simulink model "NDT_Localization"  (R2022a)
settings: Solver=FixedStepAuto  StartTime=0.0  StopTime=10.0  RelTol=1e-3
model workspace (MAT data in the model file):
  SL_ROS_VariableLengthArrays_MaxSizes : object (value not decoded)
undefined symbols (not defined in the file or in its folder): null
libraries: ros2lib x9, robotlib x8, simulink x1
(part 9 of 12)

== system NDT_Localization/observation_callback/check_localizer/If Action Subsystem/register_measurement_impl/If Action Subsystem/If Action Subsystem/solve/If Action Subsystem1/For Iterator Subsystem/compute_next_step/If Action Subsystem1/For Iterator Subsystem/If Action Subsystem/If Action Subsystem3/If Action Subsystem/f_l/gradient_angle ==
  params : Inport
  Add : Sum
  Add{1,3..5,7} (5 alike) : Sum  Inputs=+-
  Add2 : Sum
  Add6 : Sum
  Bus Selector : BusSelector  OutputSignals=cx,sx,cy,sy,cz,sz
  Constant : Constant  Value=0.0
  Constant1 : Constant  Value=0.0
  Constant2 : Constant  Value=0.0
  Gain{,1..3} (4 alike) : Gain  Gain=-1
  Product{,2,4..5,7,9..11,14,17..20,22,24,27} (16 alike) : Product
  Product{1,3,6,8,12..13,15..16,21,23,25..26} (12 alike) : Product  Inputs=3
  ga_a : MATLAB Function  TreatAsAtomicUnit=on
  ga_b : MATLAB Function  TreatAsAtomicUnit=on
  ga_c : MATLAB Function  TreatAsAtomicUnit=on
  ga_d : MATLAB Function  TreatAsAtomicUnit=on
  ga_e : MATLAB Function  TreatAsAtomicUnit=on
  ga_f : MATLAB Function  TreatAsAtomicUnit=on
  ga_g : MATLAB Function  TreatAsAtomicUnit=on
  ga_h : MATLAB Function  TreatAsAtomicUnit=on
  ga_a_out : Outport
  ga_b_out : Outport  Port=2
  ga_c_out : Outport  Port=3
  ga_d_out : Outport  Port=4
  ga_e_out : Outport  Port=5
  ga_f_out : Outport  Port=6
  ga_g_out : Outport  Port=7
  ga_h_out : Outport  Port=8
  wires:
  params/1 -> Bus Selector/1
  Bus Selector/1 -> Product1/1, Product16/1, Product25/1, Product26/1, Product20/1, Product7/1, Product5/1, Product3/1, Gain/1  "<cx>"
  Bus Selector/2 -> Product6/1, Product12/1, Product14/1, Product21/1, Product23/1, Product27/1, Product24/1, Product8/1, Gain1/1  "<sx>"
  Bus Selector/3 -> Product12/2, Product13/2, Product15/2, Product16/2, ga_c/3(z), Product9/2, Product4/2, Gain2/1  "<cy>"
  Bus Selector/4 -> Product11/1, Product14/2, Product17/2, Product21/2, Product25/2, Product26/2, Product23/2, Product8/2, Product6/2, Product3/2, Product1/2, Gain3/1  "<cx>"
  Bus Selector/5 -> Product6/3, Product10/2, Product12/3, Product15/3, Product19/2, Product20/2, Product23/3, Product26/3, Product24/2, Product7/2, Product2/2, Product1/3  "<cx>"
  Bus Selector/6 -> Product11/2, Product13/3, Product16/3, Product18/2, Product21/3, Product22/2, Product25/3, Product27/2, Product8/3, Product5/2, Product3/3, Product/2  "<cx>"
  Gain1/1 -> Product13/1, Product9/1, Product2/1, Product/1
  Product/1 -> Add/1
  Product1/1 -> Add/2
  Product2/1 -> Add1/1
  Add/1 -> ga_a/1(x)
  Add1/1 -> ga_a/2(y)
  Gain/1 -> Product15/1, Product17/1, Product22/1, Product4/1
  Product4/1 -> ga_a/3(z)
  Product3/1 -> Add1/2
  Product6/1 -> Add2/2
  Product7/1 -> Add3/1
  Product8/1 -> Add3/2
  Product5/1 -> Add2/1
  Add2/1 -> ga_b/1(x)
  Product9/1 -> ga_b/3(z)
  Add3/1 -> ga_b/2(y)
  Product11/1 -> ga_c/2(y)
  Product10/1 -> ga_c/1(x)
  Gain2/1 -> Product18/1, Product19/1
  Gain3/1 -> Product10/1
  Product13/1 -> ga_d/2(y)
  Product12/1 -> ga_d/1(x)
  Product14/1 -> ga_d/3(z)
  Product19/1 -> ga_f/2(y)
  Constant/1 -> ga_f/3(z)
  Product18/1 -> ga_f/1(x)
  Product16/1 -> ga_e/2(y)
  Product17/1 -> ga_e/3(z)
  Product15/1 -> ga_e/1(x)
  Product21/1 -> Add4/2
  Product22/1 -> Add5/1
  Product23/1 -> Add5/2
  Product20/1 -> Add4/1
  Add5/1 -> ga_g/2(y)
  Product25/1 -> Add6/2
  Product26/1 -> Add7/1
  Product27/1 -> Add7/2
  Product24/1 -> Add6/1
  Constant1/1 -> ga_g/3(z)
  Add4/1 -> ga_g/1(x)
  Add7/1 -> ga_h/2(y)
  Add6/1 -> ga_h/1(x)
  Constant2/1 -> ga_h/3(z)
  ga_a/1(out) -> ga_a_out/1  "a"
  ga_b/1(out) -> ga_b_out/1  "b"
  ga_c/1(out) -> ga_c_out/1  "c"
  ga_d/1(out) -> ga_d_out/1  "d"
  ga_e/1(out) -> ga_e_out/1  "e"
  ga_f/1(out) -> ga_f_out/1  "f"
  ga_g/1(out) -> ga_g_out/1  "g"
  ga_h/1(out) -> ga_h_out/1  "h"

== system NDT_Localization/observation_callback/check_localizer/If Action Subsystem/register_measurement_impl/If Action Subsystem/If Action Subsystem/solve/If Action Subsystem1/For Iterator Subsystem/compute_next_step/If Action Subsystem1/For Iterator Subsystem/If Action Subsystem/If Action Subsystem3/If Action Subsystem/f_u/For Iterator Subsystem ==
  data : Inport
  myu : Inport  Port=2
  sigma : Inport  Port=3
  outlier_ratio : Inport  Port=4
  voxel_size_x : Inport  Port=5
  voxel_size_y : Inport  Port=6
  voxel_size_z : Inport  Port=7
  set_jacobian : Inport  Port=8
  set_gradient : Inport  Port=9
  Affine : MATLAB Function  TreatAsAtomicUnit=on
  Delay : Delay  DelayLength=1
  For Iterator : ForIterator  IterationSource=external
  MATLAB Function : MATLAB Function  TreatAsAtomicUnit=on
  Width : Width
  gradient_jaco : Subsystem
  make_c_param : Subsystem
  make_d_param : Subsystem
  score : Subsystem
  score_out : Outport
  jacobian_out : Outport  Port=2
  wires:
  make_c_param/1(c1) -> make_d_param/1(c1)
  voxel_size_z/1 -> make_c_param/4(voxel_size_z)
  outlier_ratio/1 -> make_c_param/1(outlier_ratio)
  make_d_param/2(d2) -> gradient_jaco/9(d2), score/6(d2)
  voxel_size_y/1 -> make_c_param/3(voxel_size_y)
  make_c_param/2(c2) -> make_d_param/2(c2)
  voxel_size_x/1 -> make_c_param/2(voxel_size_x)
  make_d_param/1(d1) -> score/5(d1), gradient_jaco/8(d1)
  Width/1 -> For Iterator/1
  For Iterator/1 -> gradient_jaco/3(index), MATLAB Function/2(index)
  MATLAB Function/1(pt) -> Affine/1(u)
  Affine/1(out) -> score/4(x), gradient_jaco/4(data)
  sigma/1 -> score/2(sigma), gradient_jaco/5(sigma)
  myu/1 -> gradient_jaco/6(myu), score/3(myu)
  score/1(p) -> score_out/1, Delay/1
  Delay/1 -> score/1(score)
  set_jacobian/1 -> gradient_jaco/1(set_jacobian)
  gradient_jaco/1(Out1) -> jacobian_out/1
  set_gradient/1 -> gradient_jaco/2(set_gradient)
  data/1 -> gradient_jaco/7(x), MATLAB Function/1(data), Width/1

== system NDT_Localization/observation_callback/check_localizer/If Action Subsystem/register_measurement_impl/If Action Subsystem/If Action Subsystem/solve/If Action Subsystem1/For Iterator Subsystem/compute_next_step/If Action Subsystem1/For Iterator Subsystem/If Action Subsystem/If Action Subsystem3/If Action Subsystem/f_u/angle_params ==
  pose : Inport
  Bus Creator : BusCreator  Inputs=6
  If : If  NumInputs=2  IfExpression=u1 > u2
  If Action Subsystem : Subsystem  TreatAsAtomicUnit=on
  If Action Subsystem1 : Subsystem  TreatAsAtomicUnit=on
  If Action Subsystem2 : Subsystem  TreatAsAtomicUnit=on
  If Action Subsystem3 : Subsystem  TreatAsAtomicUnit=on
  If Action Subsystem4 : Subsystem  TreatAsAtomicUnit=on
  If Action Subsystem5 : Subsystem  TreatAsAtomicUnit=on
  If1 : If  NumInputs=2  IfExpression=u1 > u2
  If2 : If  NumInputs=2  IfExpression=u1 > u2
  MATLAB Function : MATLAB Function  TreatAsAtomicUnit=on
  Merge{,1..5} (6 alike) : Merge
  approx_thresh : Constant  Value=0.00010
  params : Outport
  wires:
  pose/1 -> MATLAB Function/1(u)
  MATLAB Function/1(x) -> If/2, If Action Subsystem1/1(x)
  MATLAB Function/3(z) -> If2/2, If Action Subsystem5/1(z)
  MATLAB Function/2(y) -> If Action Subsystem3/1(y), If1/2
  If Action Subsystem1/1(Out1) -> Merge/2
  If Action Subsystem1/2(Out2) -> Merge1/2
  If Action Subsystem3/1(Out1) -> Merge2/2
  If Action Subsystem3/2(Out2) -> Merge3/2
  If Action Subsystem5/1(Out1) -> Merge4/2
  If Action Subsystem5/2(Out2) -> Merge5/2
  approx_thresh/1 -> If2/1, If1/1, If/1
  If/1 -> If Action Subsystem/Action
  If/2 -> If Action Subsystem1/Action
  If1/1 -> If Action Subsystem2/Action
  If1/2 -> If Action Subsystem3/Action
  If2/2 -> If Action Subsystem5/Action
  If2/1 -> If Action Subsystem4/Action
  If Action Subsystem/1(Out1) -> Merge/1
  If Action Subsystem/2(Out2) -> Merge1/1
  If Action Subsystem2/1(Out1) -> Merge2/1
  If Action Subsystem2/2(Out2) -> Merge3/1
  If Action Subsystem4/1(Out1) -> Merge4/1
  If Action Subsystem4/2(Out2) -> Merge5/1
  Bus Creator/1 -> params/1
  Merge/1 -> Bus Creator/1  "cx"
  Merge1/1 -> Bus Creator/2  "sx"
  Merge2/1 -> Bus Creator/3  "cy"
  Merge3/1 -> Bus Creator/4  "sy"
  Merge4/1 -> Bus Creator/5  "cz"
  Merge5/1 -> Bus Creator/6  "sz"

== system NDT_Localization/observation_callback/check_localizer/If Action Subsystem/register_measurement_impl/If Action Subsystem/If Action Subsystem/solve/If Action Subsystem1/For Iterator Subsystem/compute_next_step/If Action Subsystem1/For Iterator Subsystem/If Action Subsystem/If Action Subsystem3/If Action Subsystem/f_u/gradient_angle ==
  params : Inport
  Add : Sum
  Add{1,3..5,7} (5 alike) : Sum  Inputs=+-
  Add2 : Sum
  Add6 : Sum
  Bus Selector : BusSelector  OutputSignals=cx,sx,cy,sy,cz,sz
  Constant : Constant  Value=0.0
  Constant1 : Constant  Value=0.0
  Constant2 : Constant  Value=0.0
  Gain{,1..3} (4 alike) : Gain  Gain=-1
  Product{,2,4..5,7,9..11,14,17..20,22,24,27} (16 alike) : Product
  Product{1,3,6,8,12..13,15..16,21,23,25..26} (12 alike) : Product  Inputs=3
  ga_a : MATLAB Function  TreatAsAtomicUnit=on
  ga_b : MATLAB Function  TreatAsAtomicUnit=on
  ga_c : MATLAB Function  TreatAsAtomicUnit=on
  ga_d : MATLAB Function  TreatAsAtomicUnit=on
  ga_e : MATLAB Function  TreatAsAtomicUnit=on
  ga_f : MATLAB Function  TreatAsAtomicUnit=on
  ga_g : MATLAB Function  TreatAsAtomicUnit=on
  ga_h : MATLAB Function  TreatAsAtomicUnit=on
  ga_a_out : Outport
  ga_b_out : Outport  Port=2
  ga_c_out : Outport  Port=3
  ga_d_out : Outport  Port=4
  ga_e_out : Outport  Port=5
  ga_f_out : Outport  Port=6
  ga_g_out : Outport  Port=7
  ga_h_out : Outport  Port=8
  wires:
  params/1 -> Bus Selector/1
  Bus Selector/1 -> Product1/1, Product16/1, Product25/1, Product26/1, Product20/1, Product7/1, Product5/1, Product3/1, Gain/1  "<cx>"
  Bus Selector/2 -> Product6/1, Product12/1, Product14/1, Product21/1, Product23/1, Product27/1, Product24/1, Product8/1, Gain1/1  "<sx>"
  Bus Selector/3 -> Product12/2, Product13/2, Product15/2, Product16/2, ga_c/3(z), Product9/2, Product4/2, Gain2/1  "<cy>"
  Bus Selector/4 -> Product11/1, Product14/2, Product17/2, Product21/2, Product25/2, Product26/2, Product23/2, Product8/2, Product6/2, Product3/2, Product1/2, Gain3/1  "<cx>"
  Bus Selector/5 -> Product6/3, Product10/2, Product12/3, Product15/3, Product19/2, Product20/2, Product23/3, Product26/3, Product24/2, Product7/2, Product2/2, Product1/3  "<cx>"
  Bus Selector/6 -> Product11/2, Product13/3, Product16/3, Product18/2, Product21/3, Product22/2, Product25/3, Product27/2, Product8/3, Product5/2, Product3/3, Product/2  "<cx>"
  Gain1/1 -> Product13/1, Product9/1, Product2/1, Product/1
  Product/1 -> Add/1
  Product1/1 -> Add/2
  Product2/1 -> Add1/1
  Add/1 -> ga_a/1(x)
  Add1/1 -> ga_a/2(y)
  Gain/1 -> Product15/1, Product17/1, Product22/1, Product4/1
  Product4/1 -> ga_a/3(z)
  Product3/1 -> Add1/2
  Product6/1 -> Add2/2
  Product7/1 -> Add3/1
  Product8/1 -> Add3/2
  Product5/1 -> Add2/1
  Add2/1 -> ga_b/1(x)
  Product9/1 -> ga_b/3(z)
  Add3/1 -> ga_b/2(y)
  Product11/1 -> ga_c/2(y)
  Product10/1 -> ga_c/1(x)
  Gain2/1 -> Product18/1, Product19/1
  Gain3/1 -> Product10/1
  Product13/1 -> ga_d/2(y)
  Product12/1 -> ga_d/1(x)
  Product14/1 -> ga_d/3(z)
  Product19/1 -> ga_f/2(y)
  Constant/1 -> ga_f/3(z)
  Product18/1 -> ga_f/1(x)
  Product16/1 -> ga_e/2(y)
  Product17/1 -> ga_e/3(z)
  Product15/1 -> ga_e/1(x)
  Product21/1 -> Add4/2
  Product22/1 -> Add5/1
  Product23/1 -> Add5/2
  Product20/1 -> Add4/1
  Add5/1 -> ga_g/2(y)
  Product25/1 -> Add6/2
  Product26/1 -> Add7/1
  Product27/1 -> Add7/2
  Product24/1 -> Add6/1
  Constant1/1 -> ga_g/3(z)
  Add4/1 -> ga_g/1(x)
  Add7/1 -> ga_h/2(y)
  Add6/1 -> ga_h/1(x)
  Constant2/1 -> ga_h/3(z)
  ga_a/1(out) -> ga_a_out/1  "a"
  ga_b/1(out) -> ga_b_out/1  "b"
  ga_c/1(out) -> ga_c_out/1  "c"
  ga_d/1(out) -> ga_d_out/1  "d"
  ga_e/1(out) -> ga_e_out/1  "e"
  ga_f/1(out) -> ga_f_out/1  "f"
  ga_g/1(out) -> ga_g_out/1  "g"
  ga_h/1(out) -> ga_h_out/1  "h"

== system NDT_Localization/observation_callback/check_localizer/If Action Subsystem/register_measurement_impl/If Action Subsystem/If Action Subsystem/solve/If Action Subsystem1/For Iterator Subsystem/compute_next_step/If Action Subsystem1/For Iterator Subsystem/If Action Subsystem/If Action Subsystem3/phi_t/For Iterator Subsystem/gradient_jaco ==
  set_jacobian : Inport
  set_gradient : Inport  Port=2
  index : Inport  Port=3
  data : Inport  Port=4
  sigma : Inport  Port=5
  myu : Inport  Port=6
  x : Inport  Port=7
  d1 : Inport  Port=8
  d2 : Inport  Port=9
  Add : Sum  Inputs=+-
  Constant : Constant  Value=-2
  Divide1 : Product  Inputs=*/
  Math Function : Math
  Math Function1 : Math  Operator=transpose
  Math Function2 : Math  Operator=reciprocal
  Product : Product  Inputs=4
  Product1 : Product  Inputs=3  Multiplication=Matrix(*)
  Product2 : Product
  Product3 : Product
  Product4 : Product  Multiplication=Matrix(*)
  gradient_col : MATLAB Function  TreatAsAtomicUnit=on
  jaco_add : MATLAB Function  TreatAsAtomicUnit=on
  Out1 : Outport
  wires:
  myu/1 -> Add/2
  Constant/1 -> Divide1/2
  Math Function1/1 -> Product1/1
  Divide1/1 -> Product2/1
  d2/1 -> Divide1/1, Product/3  "d2"
  Math Function2/1 -> Product3/2, Product1/2  "inv_cov"
  Product1/1 -> Product2/2
  d1/1 -> Product/2  "d1"
  x/1 -> Add/1
  Math Function/1 -> Product/4
  Product2/1 -> Math Function/1
  Add/1 -> Product1/3, Math Function1/1  "x-myu"
  sigma/1 -> Math Function2/1
  Product/1 -> jaco_add/3(num)
  index/1 -> jaco_add/2(index), gradient_col/1(index)
  jaco_add/1(jacobian) -> Out1/1
  set_jacobian/1 -> jaco_add/1("jacobian ")
  set_gradient/1 -> gradient_col/2(gradient)
  gradient_col/1(y) -> Product3/1
  data/1 -> Product4/1
  Product3/1 -> Product4/2
  Product4/1 -> Product/1

== system NDT_Localization/observation_callback/check_localizer/If Action Subsystem/register_measurement_impl/If Action Subsystem/If Action Subsystem/solve/If Action Subsystem1/For Iterator Subsystem/compute_next_step/If Action Subsystem1/For Iterator Subsystem/If Action Subsystem/If Action Subsystem3/phi_t/For Iterator Subsystem/make_c_param ==
  outlier_ratio : Inport
  voxel_size_x : Inport  Port=2
  voxel_size_y : Inport  Port=3
  voxel_size_z : Inport  Port=4
  Constant : Constant
  Divide : Product  Inputs=*/
  Gain : Gain  Gain=10
  Product : Product  Inputs=3
  Subtract : Sum  Inputs=+-
  c1 : Outport
  c2 : Outport  Port=2
  wires:
  Constant/1 -> Subtract/1
  outlier_ratio/1 -> Divide/1, Subtract/2
  Subtract/1 -> Gain/1
  Gain/1 -> c1/1
  Product/1 -> Divide/2
  Divide/1 -> c2/1
  voxel_size_y/1 -> Product/2
  voxel_size_z/1 -> Product/3
  voxel_size_x/1 -> Product/1

== system NDT_Localization/observation_callback/check_localizer/If Action Subsystem/register_measurement_impl/If Action Subsystem/If Action Subsystem/solve/If Action Subsystem1/For Iterator Subsystem/compute_next_step/If Action Subsystem1/For Iterator Subsystem/If Action Subsystem/If Action Subsystem3/phi_t/For Iterator Subsystem/make_d_param ==
  c1 : Inport
  c2 : Inport  Port=2
  Add1 : Sum
  Add2 : Sum  Inputs=-+
  Add3 : Sum
  Add4 : Sum  Inputs=+-
  Constant : Constant  Value=-2
  Constant1 : Constant  Value=-0.5
  Divide : Product  Inputs=*/
  Math Function{3..4,6..7} (4 alike) : Math  Operator=log
  Math Function5 : Math
  Product3 : Product
  Product4 : Product
  d1 : Outport
  d2 : Outport  Port=2
  wires:
  Add2/1 -> Divide/2, d1/1  "d1"
  Math Function4/1 -> Add4/1, Add2/2  "-d3"
  Product4/1 -> Add3/1
  Add3/1 -> Math Function6/1
  c1/1 -> Product4/1, Add1/1
  Constant/1 -> Product3/2
  Constant1/1 -> Math Function5/1
  Product3/1 -> d2/1  "d2"
  Math Function5/1 -> Product4/2
  Math Function7/1 -> Product3/1
  Divide/1 -> Math Function7/1
  Math Function6/1 -> Add4/2
  c2/1 -> Add3/2, Math Function4/1, Add1/2
  Add4/1 -> Divide/1
  Add1/1 -> Math Function3/1
  Math Function3/1 -> Add2/1

== system NDT_Localization/observation_callback/check_localizer/If Action Subsystem/register_measurement_impl/If Action Subsystem/If Action Subsystem/solve/If Action Subsystem1/For Iterator Subsystem/compute_next_step/If Action Subsystem1/For Iterator Subsystem/If Action Subsystem/If Action Subsystem3/phi_t/For Iterator Subsystem/score ==
  score : Inport
  sigma : Inport  Port=2
  myu : Inport  Port=3
  x : Inport  Port=4
  d1 : Inport  Port=5
  d2 : Inport  Port=6
  Add : Sum  Inputs=+-
  Add1 : Sum
  Constant : Constant  Value=-2
  Divide1 : Product  Inputs=*/
  Gain : Gain  Gain=-1
  Math Function : Math
  Math Function1 : Math  Operator=transpose
  Math Function2 : Math  Operator=reciprocal
  Product : Product
  Product1 : Product  Inputs=3  Multiplication=Matrix(*)
  Product2 : Product
  p : Outport
  wires:
  sigma/1 -> Math Function2/1
  Math Function/1 -> Product/2
  Gain/1 -> Product/1  "-d1"
  myu/1 -> Add/2
  x/1 -> Add/1
  Product2/1 -> Math Function/1
  Add/1 -> Product1/3, Math Function1/1  "x-myu"
  Product/1 -> Add1/2
  Math Function1/1 -> Product1/1
  Product1/1 -> Product2/2
  Math Function2/1 -> Product1/2
  Constant/1 -> Divide1/2
  Divide1/1 -> Product2/1
  d2/1 -> Divide1/1  "d2"
  d1/1 -> Gain/1
  Add1/1 -> p/1
  score/1 -> Add1/1

== system NDT_Localization/observation_callback/check_localizer/If Action Subsystem/register_measurement_impl/If Action Subsystem/If Action Subsystem/solve/If Action Subsystem1/For Iterator Subsystem/compute_next_step/If Action Subsystem1/For Iterator Subsystem/If Action Subsystem/If Action Subsystem3/phi_t/angle_params/If Action Subsystem ==
  Action Port : ActionPort
  Constant : Constant
  Constant1 : Constant  Value=0
  Out1 : Outport
  Out2 : Outport  Port=2
  wires:
  Constant/1 -> Out1/1
  Constant1/1 -> Out2/1

== system NDT_Localization/observation_callback/check_localizer/If Action Subsystem/register_measurement_impl/If Action Subsystem/If Action Subsystem/solve/If Action Subsystem1/For Iterator Subsystem/compute_next_step/If Action Subsystem1/For Iterator Subsystem/If Action Subsystem/If Action Subsystem3/phi_t/angle_params/If Action Subsystem1 ==
  x : Inport
  Action Port : ActionPort
  Trigonometric Function : Trigonometry  Operator=cos
  Trigonometric Function1 : Trigonometry
  Out1 : Outport
  Out2 : Outport  Port=2
  wires:
  x/1 -> Trigonometric Function1/1, Trigonometric Function/1
  Trigonometric Function1/1 -> Out2/1
  Trigonometric Function/1 -> Out1/1

== system NDT_Localization/observation_callback/check_localizer/If Action Subsystem/register_measurement_impl/If Action Subsystem/If Action Subsystem/solve/If Action Subsystem1/For Iterator Subsystem/compute_next_step/If Action Subsystem1/For Iterator Subsystem/If Action Subsystem/If Action Subsystem3/phi_t/angle_params/If Action Subsystem2 ==
  Action Port : ActionPort
  Constant : Constant
  Constant1 : Constant  Value=0
  Out1 : Outport
  Out2 : Outport  Port=2
  wires:
  Constant/1 -> Out1/1
  Constant1/1 -> Out2/1

== system NDT_Localization/observation_callback/check_localizer/If Action Subsystem/register_measurement_impl/If Action Subsystem/If Action Subsystem/solve/If Action Subsystem1/For Iterator Subsystem/compute_next_step/If Action Subsystem1/For Iterator Subsystem/If Action Subsystem/If Action Subsystem3/phi_t/angle_params/If Action Subsystem3 ==
  y : Inport
  Action Port : ActionPort
  Trigonometric Function : Trigonometry  Operator=cos
  Trigonometric Function1 : Trigonometry
  Out1 : Outport
  Out2 : Outport  Port=2
  wires:
  Trigonometric Function/1 -> Out1/1
  Trigonometric Function1/1 -> Out2/1
  y/1 -> Trigonometric Function1/1, Trigonometric Function/1

== system NDT_Localization/observation_callback/check_localizer/If Action Subsystem/register_measurement_impl/If Action Subsystem/If Action Subsystem/solve/If Action Subsystem1/For Iterator Subsystem/compute_next_step/If Action Subsystem1/For Iterator Subsystem/If Action Subsystem/If Action Subsystem3/phi_t/angle_params/If Action Subsystem4 ==
  Action Port : ActionPort
  Constant : Constant
  Constant1 : Constant  Value=0
  Out1 : Outport
  Out2 : Outport  Port=2
  wires:
  Constant/1 -> Out1/1
  Constant1/1 -> Out2/1

== system NDT_Localization/observation_callback/check_localizer/If Action Subsystem/register_measurement_impl/If Action Subsystem/If Action Subsystem/solve/If Action Subsystem1/For Iterator Subsystem/compute_next_step/If Action Subsystem1/For Iterator Subsystem/If Action Subsystem/If Action Subsystem3/phi_t/angle_params/If Action Subsystem5 ==
  z : Inport
  Action Port : ActionPort
  Trigonometric Function : Trigonometry  Operator=cos
  Trigonometric Function1 : Trigonometry
  Out1 : Outport
  Out2 : Outport  Port=2
  wires:
  Trigonometric Function1/1 -> Out2/1
  Trigonometric Function/1 -> Out1/1
  z/1 -> Trigonometric Function1/1, Trigonometric Function/1

== system NDT_Localization/observation_callback/check_localizer/If Action Subsystem/register_measurement_impl/If Action Subsystem/If Action Subsystem/solve/If Action Subsystem1/For Iterator Subsystem/compute_next_step/If Action Subsystem1/For Iterator Subsystem/If Action Subsystem/If Action Subsystem3/psi_t/initial_objective_function/For Iterator Subsystem ==
  data : Inport
  myu : Inport  Port=2
  sigma : Inport  Port=3
  outlier_ratio : Inport  Port=4
  voxel_size_x : Inport  Port=5
  voxel_size_y : Inport  Port=6
  voxel_size_z : Inport  Port=7
  set_jacobian : Inport  Port=8
  set_gradient : Inport  Port=9
  Affine : MATLAB Function  TreatAsAtomicUnit=on
  Delay : Delay  DelayLength=1
  For Iterator : ForIterator  IterationSource=external
  MATLAB Function : MATLAB Function  TreatAsAtomicUnit=on
  Width : Width
  gradient_jaco : Subsystem
  make_c_param : Subsystem
  make_d_param : Subsystem
  score : Subsystem
  score_out : Outport
  jacobian_out : Outport  Port=2
  wires:
  make_c_param/1(c1) -> make_d_param/1(c1)
  voxel_size_z/1 -> make_c_param/4(voxel_size_z)
  outlier_ratio/1 -> make_c_param/1(outlier_ratio)
  make_d_param/2(d2) -> gradient_jaco/9(d2), score/6(d2)
  voxel_size_y/1 -> make_c_param/3(voxel_size_y)
  make_c_param/2(c2) -> make_d_param/2(c2)
  voxel_size_x/1 -> make_c_param/2(voxel_size_x)
  make_d_param/1(d1) -> score/5(d1), gradient_jaco/8(d1)
  Width/1 -> For Iterator/1
  For Iterator/1 -> gradient_jaco/3(index), MATLAB Function/2(index)
  MATLAB Function/1(pt) -> Affine/1(u)
  Affine/1(out) -> score/4(x), gradient_jaco/4(data)
  sigma/1 -> score/2(sigma), gradient_jaco/5(sigma)
  myu/1 -> gradient_jaco/6(myu), score/3(myu)
  score/1(p) -> score_out/1, Delay/1
  Delay/1 -> score/1(score)
  set_jacobian/1 -> gradient_jaco/1(set_jacobian)
  gradient_jaco/1(Out1) -> jacobian_out/1
  set_gradient/1 -> gradient_jaco/2(set_gradient)
  data/1 -> gradient_jaco/7(x), MATLAB Function/1(data), Width/1

== system NDT_Localization/observation_callback/check_localizer/If Action Subsystem/register_measurement_impl/If Action Subsystem/If Action Subsystem/solve/If Action Subsystem1/For Iterator Subsystem/compute_next_step/If Action Subsystem1/For Iterator Subsystem/If Action Subsystem/If Action Subsystem3/psi_t/initial_objective_function/angle_params ==
  pose : Inport
  Bus Creator : BusCreator  Inputs=6
  If : If  NumInputs=2  IfExpression=u1 > u2
  If Action Subsystem : Subsystem  TreatAsAtomicUnit=on
  If Action Subsystem1 : Subsystem  TreatAsAtomicUnit=on
  If Action Subsystem2 : Subsystem  TreatAsAtomicUnit=on
  If Action Subsystem3 : Subsystem  TreatAsAtomicUnit=on
  If Action Subsystem4 : Subsystem  TreatAsAtomicUnit=on
  If Action Subsystem5 : Subsystem  TreatAsAtomicUnit=on
  If1 : If  NumInputs=2  IfExpression=u1 > u2
  If2 : If  NumInputs=2  IfExpression=u1 > u2
  MATLAB Function : MATLAB Function  TreatAsAtomicUnit=on
  Merge{,1..5} (6 alike) : Merge
  approx_thresh : Constant  Value=0.00010
  params : Outport
  wires:
  pose/1 -> MATLAB Function/1(u)
  MATLAB Function/1(x) -> If/2, If Action Subsystem1/1(x)
  MATLAB Function/3(z) -> If2/2, If Action Subsystem5/1(z)
  MATLAB Function/2(y) -> If Action Subsystem3/1(y), If1/2
  If Action Subsystem1/1(Out1) -> Merge/2
  If Action Subsystem1/2(Out2) -> Merge1/2
  If Action Subsystem3/1(Out1) -> Merge2/2
  If Action Subsystem3/2(Out2) -> Merge3/2
  If Action Subsystem5/1(Out1) -> Merge4/2
  If Action Subsystem5/2(Out2) -> Merge5/2
  approx_thresh/1 -> If2/1, If1/1, If/1
  If/1 -> If Action Subsystem/Action
  If/2 -> If Action Subsystem1/Action
  If1/1 -> If Action Subsystem2/Action
  If1/2 -> If Action Subsystem3/Action
  If2/2 -> If Action Subsystem5/Action
  If2/1 -> If Action Subsystem4/Action
  If Action Subsystem/1(Out1) -> Merge/1
  If Action Subsystem/2(Out2) -> Merge1/1
  If Action Subsystem2/1(Out1) -> Merge2/1
  If Action Subsystem2/2(Out2) -> Merge3/1
  If Action Subsystem4/1(Out1) -> Merge4/1
  If Action Subsystem4/2(Out2) -> Merge5/1
  Bus Creator/1 -> params/1
  Merge/1 -> Bus Creator/1  "cx"
  Merge1/1 -> Bus Creator/2  "sx"
  Merge2/1 -> Bus Creator/3  "cy"
  Merge3/1 -> Bus Creator/4  "sy"
  Merge4/1 -> Bus Creator/5  "cz"
  Merge5/1 -> Bus Creator/6  "sz"

== system NDT_Localization/observation_callback/check_localizer/If Action Subsystem/register_measurement_impl/If Action Subsystem/If Action Subsystem/solve/If Action Subsystem1/For Iterator Subsystem/compute_next_step/If Action Subsystem1/For Iterator Subsystem/If Action Subsystem/If Action Subsystem3/psi_t/initial_objective_function/gradient_angle ==
  params : Inport
  Add : Sum
  Add{1,3..5,7} (5 alike) : Sum  Inputs=+-
  Add2 : Sum
  Add6 : Sum
  Bus Selector : BusSelector  OutputSignals=cx,sx,cy,sy,cz,sz
  Constant : Constant  Value=0.0
  Constant1 : Constant  Value=0.0
  Constant2 : Constant  Value=0.0
  Gain{,1..3} (4 alike) : Gain  Gain=-1
  Product{,2,4..5,7,9..11,14,17..20,22,24,27} (16 alike) : Product
  Product{1,3,6,8,12..13,15..16,21,23,25..26} (12 alike) : Product  Inputs=3
  ga_a : MATLAB Function  TreatAsAtomicUnit=on
  ga_b : MATLAB Function  TreatAsAtomicUnit=on
  ga_c : MATLAB Function  TreatAsAtomicUnit=on
  ga_d : MATLAB Function  TreatAsAtomicUnit=on
  ga_e : MATLAB Function  TreatAsAtomicUnit=on
  ga_f : MATLAB Function  TreatAsAtomicUnit=on
  ga_g : MATLAB Function  TreatAsAtomicUnit=on
  ga_h : MATLAB Function  TreatAsAtomicUnit=on
  ga_a_out : Outport
  ga_b_out : Outport  Port=2
  ga_c_out : Outport  Port=3
  ga_d_out : Outport  Port=4
  ga_e_out : Outport  Port=5
  ga_f_out : Outport  Port=6
  ga_g_out : Outport  Port=7
  ga_h_out : Outport  Port=8
  wires:
  params/1 -> Bus Selector/1
  Bus Selector/1 -> Product1/1, Product16/1, Product25/1, Product26/1, Product20/1, Product7/1, Product5/1, Product3/1, Gain/1  "<cx>"
  Bus Selector/2 -> Product6/1, Product12/1, Product14/1, Product21/1, Product23/1, Product27/1, Product24/1, Product8/1, Gain1/1  "<sx>"
  Bus Selector/3 -> Product12/2, Product13/2, Product15/2, Product16/2, ga_c/3(z), Product9/2, Product4/2, Gain2/1  "<cy>"
  Bus Selector/4 -> Product11/1, Product14/2, Product17/2, Product21/2, Product25/2, Product26/2, Product23/2, Product8/2, Product6/2, Product3/2, Product1/2, Gain3/1  "<cx>"
  Bus Selector/5 -> Product6/3, Product10/2, Product12/3, Product15/3, Product19/2, Product20/2, Product23/3, Product26/3, Product24/2, Product7/2, Product2/2, Product1/3  "<cx>"
  Bus Selector/6 -> Product11/2, Product13/3, Product16/3, Product18/2, Product21/3, Product22/2, Product25/3, Product27/2, Product8/3, Product5/2, Product3/3, Product/2  "<cx>"
  Gain1/1 -> Product13/1, Product9/1, Product2/1, Product/1
  Product/1 -> Add/1
  Product1/1 -> Add/2
  Product2/1 -> Add1/1
  Add/1 -> ga_a/1(x)
  Add1/1 -> ga_a/2(y)
  Gain/1 -> Product15/1, Product17/1, Product22/1, Product4/1
  Product4/1 -> ga_a/3(z)
  Product3/1 -> Add1/2
  Product6/1 -> Add2/2
  Product7/1 -> Add3/1
  Product8/1 -> Add3/2
  Product5/1 -> Add2/1
  Add2/1 -> ga_b/1(x)
  Product9/1 -> ga_b/3(z)
  Add3/1 -> ga_b/2(y)
  Product11/1 -> ga_c/2(y)
  Product10/1 -> ga_c/1(x)
  Gain2/1 -> Product18/1, Product19/1
  Gain3/1 -> Product10/1
  Product13/1 -> ga_d/2(y)
  Product12/1 -> ga_d/1(x)
  Product14/1 -> ga_d/3(z)
  Product19/1 -> ga_f/2(y)
  Constant/1 -> ga_f/3(z)
  Product18/1 -> ga_f/1(x)
  Product16/1 -> ga_e/2(y)
  Product17/1 -> ga_e/3(z)
  Product15/1 -> ga_e/1(x)
  Product21/1 -> Add4/2
  Product22/1 -> Add5/1
  Product23/1 -> Add5/2
  Product20/1 -> Add4/1
  Add5/1 -> ga_g/2(y)
  Product25/1 -> Add6/2
  Product26/1 -> Add7/1
  Product27/1 -> Add7/2
  Product24/1 -> Add6/1
  Constant1/1 -> ga_g/3(z)
  Add4/1 -> ga_g/1(x)
  Add7/1 -> ga_h/2(y)
  Add6/1 -> ga_h/1(x)
  Constant2/1 -> ga_h/3(z)
  ga_a/1(out) -> ga_a_out/1  "a"
  ga_b/1(out) -> ga_b_out/1  "b"
  ga_c/1(out) -> ga_c_out/1  "c"
  ga_d/1(out) -> ga_d_out/1  "d"
  ga_e/1(out) -> ga_e_out/1  "e"
  ga_f/1(out) -> ga_f_out/1  "f"
  ga_g/1(out) -> ga_g_out/1  "g"
  ga_h/1(out) -> ga_h_out/1  "h"

== system NDT_Localization/observation_callback/check_localizer/If Action Subsystem/register_measurement_impl/If Action Subsystem/If Action Subsystem/solve/If Action Subsystem1/For Iterator Subsystem/compute_next_step/If Action Subsystem1/For Iterator Subsystem/If Action Subsystem/If Action Subsystem3/psi_t/objective_function/For Iterator Subsystem ==
  data : Inport
  myu : Inport  Port=2
  sigma : Inport  Port=3
  outlier_ratio : Inport  Port=4
  voxel_size_x : Inport  Port=5
  voxel_size_y : Inport  Port=6
  voxel_size_z : Inport  Port=7
  set_jacobian : Inport  Port=8
  set_gradient : Inport  Port=9
  Affine : MATLAB Function  TreatAsAtomicUnit=on
  Delay : Delay  DelayLength=1
  For Iterator : ForIterator  IterationSource=external
  MATLAB Function : MATLAB Function  TreatAsAtomicUnit=on
  Width : Width
  gradient_jaco : Subsystem
  make_c_param : Subsystem
  make_d_param : Subsystem
  score : Subsystem
  score_out : Outport
  jacobian_out : Outport  Port=2
  wires:
  make_c_param/1(c1) -> make_d_param/1(c1)
  voxel_size_z/1 -> make_c_param/4(voxel_size_z)
  outlier_ratio/1 -> make_c_param/1(outlier_ratio)
  make_d_param/2(d2) -> gradient_jaco/9(d2), score/6(d2)
  voxel_size_y/1 -> make_c_param/3(voxel_size_y)
  make_c_param/2(c2) -> make_d_param/2(c2)
  voxel_size_x/1 -> make_c_param/2(voxel_size_x)
  make_d_param/1(d1) -> score/5(d1), gradient_jaco/8(d1)
  Width/1 -> For Iterator/1
  For Iterator/1 -> gradient_jaco/3(index), MATLAB Function/2(index)
  MATLAB Function/1(pt) -> Affine/1(u)
  Affine/1(out) -> score/4(x), gradient_jaco/4(data)
  sigma/1 -> score/2(sigma), gradient_jaco/5(sigma)
  myu/1 -> gradient_jaco/6(myu), score/3(myu)
  score/1(p) -> score_out/1, Delay/1
  Delay/1 -> score/1(score)
  set_jacobian/1 -> gradient_jaco/1(set_jacobian)
  gradient_jaco/1(Out1) -> jacobian_out/1
  set_gradient/1 -> gradient_jaco/2(set_gradient)
  data/1 -> gradient_jaco/7(x), MATLAB Function/1(data), Width/1

== system NDT_Localization/observation_callback/check_localizer/If Action Subsystem/register_measurement_impl/If Action Subsystem/If Action Subsystem/solve/If Action Subsystem1/For Iterator Subsystem/compute_next_step/If Action Subsystem1/For Iterator Subsystem/If Action Subsystem/If Action Subsystem3/psi_t/objective_function/angle_params ==
  pose : Inport
  Bus Creator : BusCreator  Inputs=6
  If : If  NumInputs=2  IfExpression=u1 > u2
  If Action Subsystem : Subsystem  TreatAsAtomicUnit=on
  If Action Subsystem1 : Subsystem  TreatAsAtomicUnit=on
  If Action Subsystem2 : Subsystem  TreatAsAtomicUnit=on
  If Action Subsystem3 : Subsystem  TreatAsAtomicUnit=on
  If Action Subsystem4 : Subsystem  TreatAsAtomicUnit=on
  If Action Subsystem5 : Subsystem  TreatAsAtomicUnit=on
  If1 : If  NumInputs=2  IfExpression=u1 > u2
  If2 : If  NumInputs=2  IfExpression=u1 > u2
  MATLAB Function : MATLAB Function  TreatAsAtomicUnit=on
  Merge{,1..5} (6 alike) : Merge
  approx_thresh : Constant  Value=0.00010
  params : Outport
  wires:
  pose/1 -> MATLAB Function/1(u)
  MATLAB Function/1(x) -> If/2, If Action Subsystem1/1(x)
  MATLAB Function/3(z) -> If2/2, If Action Subsystem5/1(z)
  MATLAB Function/2(y) -> If Action Subsystem3/1(y), If1/2
  If Action Subsystem1/1(Out1) -> Merge/2
  If Action Subsystem1/2(Out2) -> Merge1/2
  If Action Subsystem3/1(Out1) -> Merge2/2
  If Action Subsystem3/2(Out2) -> Merge3/2
  If Action Subsystem5/1(Out1) -> Merge4/2
  If Action Subsystem5/2(Out2) -> Merge5/2
  approx_thresh/1 -> If2/1, If1/1, If/1
  If/1 -> If Action Subsystem/Action
  If/2 -> If Action Subsystem1/Action
  If1/1 -> If Action Subsystem2/Action
  If1/2 -> If Action Subsystem3/Action
  If2/2 -> If Action Subsystem5/Action
  If2/1 -> If Action Subsystem4/Action
  If Action Subsystem/1(Out1) -> Merge/1
  If Action Subsystem/2(Out2) -> Merge1/1
  If Action Subsystem2/1(Out1) -> Merge2/1
  If Action Subsystem2/2(Out2) -> Merge3/1
  If Action Subsystem4/1(Out1) -> Merge4/1
  If Action Subsystem4/2(Out2) -> Merge5/1
  Bus Creator/1 -> params/1
  Merge/1 -> Bus Creator/1  "cx"
  Merge1/1 -> Bus Creator/2  "sx"
  Merge2/1 -> Bus Creator/3  "cy"
  Merge3/1 -> Bus Creator/4  "sy"
  Merge4/1 -> Bus Creator/5  "cz"
  Merge5/1 -> Bus Creator/6  "sz"

== system NDT_Localization/observation_callback/check_localizer/If Action Subsystem/register_measurement_impl/If Action Subsystem/If Action Subsystem/solve/If Action Subsystem1/For Iterator Subsystem/compute_next_step/If Action Subsystem1/For Iterator Subsystem/If Action Subsystem/If Action Subsystem3/psi_t/objective_function/gradient_angle ==
  params : Inport
  Add : Sum
  Add{1,3..5,7} (5 alike) : Sum  Inputs=+-
  Add2 : Sum
  Add6 : Sum
  Bus Selector : BusSelector  OutputSignals=cx,sx,cy,sy,cz,sz
  Constant : Constant  Value=0.0
  Constant1 : Constant  Value=0.0
  Constant2 : Constant  Value=0.0
  Gain{,1..3} (4 alike) : Gain  Gain=-1
  Product{,2,4..5,7,9..11,14,17..20,22,24,27} (16 alike) : Product
  Product{1,3,6,8,12..13,15..16,21,23,25..26} (12 alike) : Product  Inputs=3
  ga_a : MATLAB Function  TreatAsAtomicUnit=on
  ga_b : MATLAB Function  TreatAsAtomicUnit=on
  ga_c : MATLAB Function  TreatAsAtomicUnit=on
  ga_d : MATLAB Function  TreatAsAtomicUnit=on
  ga_e : MATLAB Function  TreatAsAtomicUnit=on
  ga_f : MATLAB Function  TreatAsAtomicUnit=on
  ga_g : MATLAB Function  TreatAsAtomicUnit=on
  ga_h : MATLAB Function  TreatAsAtomicUnit=on
  ga_a_out : Outport
  ga_b_out : Outport  Port=2
  ga_c_out : Outport  Port=3
  ga_d_out : Outport  Port=4
  ga_e_out : Outport  Port=5
  ga_f_out : Outport  Port=6
  ga_g_out : Outport  Port=7
  ga_h_out : Outport  Port=8
  wires:
  params/1 -> Bus Selector/1
  Bus Selector/1 -> Product1/1, Product16/1, Product25/1, Product26/1, Product20/1, Product7/1, Product5/1, Product3/1, Gain/1  "<cx>"
  Bus Selector/2 -> Product6/1, Product12/1, Product14/1, Product21/1, Product23/1, Product27/1, Product24/1, Product8/1, Gain1/1  "<sx>"
  Bus Selector/3 -> Product12/2, Product13/2, Product15/2, Product16/2, ga_c/3(z), Product9/2, Product4/2, Gain2/1  "<cy>"
  Bus Selector/4 -> Product11/1, Product14/2, Product17/2, Product21/2, Product25/2, Product26/2, Product23/2, Product8/2, Product6/2, Product3/2, Product1/2, Gain3/1  "<cx>"
  Bus Selector/5 -> Product6/3, Product10/2, Product12/3, Product15/3, Product19/2, Product20/2, Product23/3, Product26/3, Product24/2, Product7/2, Product2/2, Product1/3  "<cx>"
  Bus Selector/6 -> Product11/2, Product13/3, Product16/3, Product18/2, Product21/3, Product22/2, Product25/3, Product27/2, Product8/3, Product5/2, Product3/3, Product/2  "<cx>"
  Gain1/1 -> Product13/1, Product9/1, Product2/1, Product/1
  Product/1 -> Add/1
  Product1/1 -> Add/2
  Product2/1 -> Add1/1
  Add/1 -> ga_a/1(x)
  Add1/1 -> ga_a/2(y)
  Gain/1 -> Product15/1, Product17/1, Product22/1, Product4/1
  Product4/1 -> ga_a/3(z)
  Product3/1 -> Add1/2
  Product6/1 -> Add2/2
  Product7/1 -> Add3/1
  Product8/1 -> Add3/2
  Product5/1 -> Add2/1
  Add2/1 -> ga_b/1(x)
  Product9/1 -> ga_b/3(z)
  Add3/1 -> ga_b/2(y)
  Product11/1 -> ga_c/2(y)
  Product10/1 -> ga_c/1(x)
  Gain2/1 -> Product18/1, Product19/1
  Gain3/1 -> Product10/1
  Product13/1 -> ga_d/2(y)
  Product12/1 -> ga_d/1(x)
  Product14/1 -> ga_d/3(z)
  Product19/1 -> ga_f/2(y)
  Constant/1 -> ga_f/3(z)
  Product18/1 -> ga_f/1(x)
  Product16/1 -> ga_e/2(y)
  Product17/1 -> ga_e/3(z)
  Product15/1 -> ga_e/1(x)
  Product21/1 -> Add4/2
  Product22/1 -> Add5/1
  Product23/1 -> Add5/2
  Product20/1 -> Add4/1
  Add5/1 -> ga_g/2(y)
  Product25/1 -> Add6/2
  Product26/1 -> Add7/1
  Product27/1 -> Add7/2
  Product24/1 -> Add6/1
  Constant1/1 -> ga_g/3(z)
  Add4/1 -> ga_g/1(x)
  Add7/1 -> ga_h/2(y)
  Add6/1 -> ga_h/1(x)
  Constant2/1 -> ga_h/3(z)
  ga_a/1(out) -> ga_a_out/1  "a"
  ga_b/1(out) -> ga_b_out/1  "b"
  ga_c/1(out) -> ga_c_out/1  "c"
  ga_d/1(out) -> ga_d_out/1  "d"
  ga_e/1(out) -> ga_e_out/1  "e"
  ga_f/1(out) -> ga_f_out/1  "f"
  ga_g/1(out) -> ga_g_out/1  "g"
  ga_h/1(out) -> ga_h_out/1  "h"

== system NDT_Localization/observation_callback/check_localizer/If Action Subsystem/register_measurement_impl/If Action Subsystem/If Action Subsystem/solve/If Action Subsystem1/For Iterator Subsystem/compute_next_step/If Action Subsystem1/For Iterator Subsystem/If Action Subsystem/If Action Subsystem3/If Action Subsystem/f_l/For Iterator Subsystem/gradient_jaco ==
  set_jacobian : Inport
  set_gradient : Inport  Port=2
  index : Inport  Port=3
  data : Inport  Port=4
  sigma : Inport  Port=5
  myu : Inport  Port=6
  x : Inport  Port=7
  d1 : Inport  Port=8
  d2 : Inport  Port=9
  Add : Sum  Inputs=+-
  Constant : Constant  Value=-2
  Divide1 : Product  Inputs=*/
  Math Function : Math
  Math Function1 : Math  Operator=transpose
  Math Function2 : Math  Operator=reciprocal
  Product : Product  Inputs=4
  Product1 : Product  Inputs=3  Multiplication=Matrix(*)
  Product2 : Product
  Product3 : Product
  Product4 : Product  Multiplication=Matrix(*)
  gradient_col : MATLAB Function  TreatAsAtomicUnit=on
  jaco_add : MATLAB Function  TreatAsAtomicUnit=on
  Out1 : Outport
  wires:
  myu/1 -> Add/2
  Constant/1 -> Divide1/2
  Math Function1/1 -> Product1/1
  Divide1/1 -> Product2/1
  d2/1 -> Divide1/1, Product/3  "d2"
  Math Function2/1 -> Product3/2, Product1/2  "inv_cov"
  Product1/1 -> Product2/2
  d1/1 -> Product/2  "d1"
  x/1 -> Add/1
  Math Function/1 -> Product/4
  Product2/1 -> Math Function/1
  Add/1 -> Product1/3, Math Function1/1  "x-myu"
  sigma/1 -> Math Function2/1
  Product/1 -> jaco_add/3(num)
  index/1 -> jaco_add/2(index), gradient_col/1(index)
  jaco_add/1(jacobian) -> Out1/1
  set_jacobian/1 -> jaco_add/1("jacobian ")
  set_gradient/1 -> gradient_col/2(gradient)
  gradient_col/1(y) -> Product3/1
  data/1 -> Product4/1
  Product3/1 -> Product4/2
  Product4/1 -> Product/1

== system NDT_Localization/observation_callback/check_localizer/If Action Subsystem/register_measurement_impl/If Action Subsystem/If Action Subsystem/solve/If Action Subsystem1/For Iterator Subsystem/compute_next_step/If Action Subsystem1/For Iterator Subsystem/If Action Subsystem/If Action Subsystem3/If Action Subsystem/f_l/For Iterator Subsystem/make_c_param ==
  outlier_ratio : Inport
  voxel_size_x : Inport  Port=2
  voxel_size_y : Inport  Port=3
  voxel_size_z : Inport  Port=4
  Constant : Constant
  Divide : Product  Inputs=*/
  Gain : Gain  Gain=10
  Product : Product  Inputs=3
  Subtract : Sum  Inputs=+-
  c1 : Outport
  c2 : Outport  Port=2
  wires:
  Constant/1 -> Subtract/1
  outlier_ratio/1 -> Divide/1, Subtract/2
  Subtract/1 -> Gain/1
  Gain/1 -> c1/1
  Product/1 -> Divide/2
  Divide/1 -> c2/1
  voxel_size_y/1 -> Product/2
  voxel_size_z/1 -> Product/3
  voxel_size_x/1 -> Product/1

== system NDT_Localization/observation_callback/check_localizer/If Action Subsystem/register_measurement_impl/If Action Subsystem/If Action Subsystem/solve/If Action Subsystem1/For Iterator Subsystem/compute_next_step/If Action Subsystem1/For Iterator Subsystem/If Action Subsystem/If Action Subsystem3/If Action Subsystem/f_l/For Iterator Subsystem/make_d_param ==
  c1 : Inport
  c2 : Inport  Port=2
  Add1 : Sum
  Add2 : Sum  Inputs=-+
  Add3 : Sum
  Add4 : Sum  Inputs=+-
  Constant : Constant  Value=-2
  Constant1 : Constant  Value=-0.5
  Divide : Product  Inputs=*/
  Math Function{3..4,6..7} (4 alike) : Math  Operator=log
  Math Function5 : Math
  Product3 : Product
  Product4 : Product
  d1 : Outport
  d2 : Outport  Port=2
  wires:
  Add2/1 -> Divide/2, d1/1  "d1"
  Math Function4/1 -> Add4/1, Add2/2  "-d3"
  Product4/1 -> Add3/1
  Add3/1 -> Math Function6/1
  c1/1 -> Product4/1, Add1/1
  Constant/1 -> Product3/2
  Constant1/1 -> Math Function5/1
  Product3/1 -> d2/1  "d2"
  Math Function5/1 -> Product4/2
  Math Function7/1 -> Product3/1
  Divide/1 -> Math Function7/1
  Math Function6/1 -> Add4/2
  c2/1 -> Add3/2, Math Function4/1, Add1/2
  Add4/1 -> Divide/1
  Add1/1 -> Math Function3/1
  Math Function3/1 -> Add2/1

== system NDT_Localization/observation_callback/check_localizer/If Action Subsystem/register_measurement_impl/If Action Subsystem/If Action Subsystem/solve/If Action Subsystem1/For Iterator Subsystem/compute_next_step/If Action Subsystem1/For Iterator Subsystem/If Action Subsystem/If Action Subsystem3/If Action Subsystem/f_l/For Iterator Subsystem/score ==
  score : Inport
  sigma : Inport  Port=2
  myu : Inport  Port=3
  x : Inport  Port=4
  d1 : Inport  Port=5
  d2 : Inport  Port=6
  Add : Sum  Inputs=+-
  Add1 : Sum
  Constant : Constant  Value=-2
  Divide1 : Product  Inputs=*/
  Gain : Gain  Gain=-1
  Math Function : Math
  Math Function1 : Math  Operator=transpose
  Math Function2 : Math  Operator=reciprocal
  Product : Product
  Product1 : Product  Inputs=3  Multiplication=Matrix(*)
  Product2 : Product
  p : Outport
  wires:
  sigma/1 -> Math Function2/1
  Math Function/1 -> Product/2
  Gain/1 -> Product/1  "-d1"
  myu/1 -> Add/2
  x/1 -> Add/1
  Product2/1 -> Math Function/1
  Add/1 -> Product1/3, Math Function1/1  "x-myu"
  Product/1 -> Add1/2
  Math Function1/1 -> Product1/1
  Product1/1 -> Product2/2
  Math Function2/1 -> Product1/2
  Constant/1 -> Divide1/2
  Divide1/1 -> Product2/1
  d2/1 -> Divide1/1  "d2"
  d1/1 -> Gain/1
  Add1/1 -> p/1
  score/1 -> Add1/1

== system NDT_Localization/observation_callback/check_localizer/If Action Subsystem/register_measurement_impl/If Action Subsystem/If Action Subsystem/solve/If Action Subsystem1/For Iterator Subsystem/compute_next_step/If Action Subsystem1/For Iterator Subsystem/If Action Subsystem/If Action Subsystem3/If Action Subsystem/f_l/angle_params/If Action Subsystem ==
  Action Port : ActionPort
  Constant : Constant
  Constant1 : Constant  Value=0
  Out1 : Outport
  Out2 : Outport  Port=2
  wires:
  Constant/1 -> Out1/1
  Constant1/1 -> Out2/1

== system NDT_Localization/observation_callback/check_localizer/If Action Subsystem/register_measurement_impl/If Action Subsystem/If Action Subsystem/solve/If Action Subsystem1/For Iterator Subsystem/compute_next_step/If Action Subsystem1/For Iterator Subsystem/If Action Subsystem/If Action Subsystem3/If Action Subsystem/f_l/angle_params/If Action Subsystem1 ==
  x : Inport
  Action Port : ActionPort
  Trigonometric Function : Trigonometry  Operator=cos
  Trigonometric Function1 : Trigonometry
  Out1 : Outport
  Out2 : Outport  Port=2
  wires:
  x/1 -> Trigonometric Function1/1, Trigonometric Function/1
  Trigonometric Function1/1 -> Out2/1
  Trigonometric Function/1 -> Out1/1

== system NDT_Localization/observation_callback/check_localizer/If Action Subsystem/register_measurement_impl/If Action Subsystem/If Action Subsystem/solve/If Action Subsystem1/For Iterator Subsystem/compute_next_step/If Action Subsystem1/For Iterator Subsystem/If Action Subsystem/If Action Subsystem3/If Action Subsystem/f_l/angle_params/If Action Subsystem2 ==
  Action Port : ActionPort
  Constant : Constant
  Constant1 : Constant  Value=0
  Out1 : Outport
  Out2 : Outport  Port=2
  wires:
  Constant/1 -> Out1/1
  Constant1/1 -> Out2/1

== system NDT_Localization/observation_callback/check_localizer/If Action Subsystem/register_measurement_impl/If Action Subsystem/If Action Subsystem/solve/If Action Subsystem1/For Iterator Subsystem/compute_next_step/If Action Subsystem1/For Iterator Subsystem/If Action Subsystem/If Action Subsystem3/If Action Subsystem/f_l/angle_params/If Action Subsystem3 ==
  y : Inport
  Action Port : ActionPort
  Trigonometric Function : Trigonometry  Operator=cos
  Trigonometric Function1 : Trigonometry
  Out1 : Outport
  Out2 : Outport  Port=2
  wires:
  Trigonometric Function/1 -> Out1/1
  Trigonometric Function1/1 -> Out2/1
  y/1 -> Trigonometric Function1/1, Trigonometric Function/1

== system NDT_Localization/observation_callback/check_localizer/If Action Subsystem/register_measurement_impl/If Action Subsystem/If Action Subsystem/solve/If Action Subsystem1/For Iterator Subsystem/compute_next_step/If Action Subsystem1/For Iterator Subsystem/If Action Subsystem/If Action Subsystem3/If Action Subsystem/f_l/angle_params/If Action Subsystem4 ==
  Action Port : ActionPort
  Constant : Constant
  Constant1 : Constant  Value=0
  Out1 : Outport
  Out2 : Outport  Port=2
  wires:
  Constant/1 -> Out1/1
  Constant1/1 -> Out2/1

== system NDT_Localization/observation_callback/check_localizer/If Action Subsystem/register_measurement_impl/If Action Subsystem/If Action Subsystem/solve/If Action Subsystem1/For Iterator Subsystem/compute_next_step/If Action Subsystem1/For Iterator Subsystem/If Action Subsystem/If Action Subsystem3/If Action Subsystem/f_l/angle_params/If Action Subsystem5 ==
  z : Inport
  Action Port : ActionPort
  Trigonometric Function : Trigonometry  Operator=cos
  Trigonometric Function1 : Trigonometry
  Out1 : Outport
  Out2 : Outport  Port=2
  wires:
  Trigonometric Function1/1 -> Out2/1
  Trigonometric Function/1 -> Out1/1
  z/1 -> Trigonometric Function1/1, Trigonometric Function/1

== system NDT_Localization/observation_callback/check_localizer/If Action Subsystem/register_measurement_impl/If Action Subsystem/If Action Subsystem/solve/If Action Subsystem1/For Iterator Subsystem/compute_next_step/If Action Subsystem1/For Iterator Subsystem/If Action Subsystem/If Action Subsystem3/If Action Subsystem/f_u/For Iterator Subsystem/gradient_jaco ==
  set_jacobian : Inport
  set_gradient : Inport  Port=2
  index : Inport  Port=3
  data : Inport  Port=4
  sigma : Inport  Port=5
  myu : Inport  Port=6
  x : Inport  Port=7
  d1 : Inport  Port=8
  d2 : Inport  Port=9
  Add : Sum  Inputs=+-
  Constant : Constant  Value=-2
  Divide1 : Product  Inputs=*/
  Math Function : Math
  Math Function1 : Math  Operator=transpose
  Math Function2 : Math  Operator=reciprocal
  Product : Product  Inputs=4
  Product1 : Product  Inputs=3  Multiplication=Matrix(*)
  Product2 : Product
  Product3 : Product
  Product4 : Product  Multiplication=Matrix(*)
  gradient_col : MATLAB Function  TreatAsAtomicUnit=on
  jaco_add : MATLAB Function  TreatAsAtomicUnit=on
  Out1 : Outport
  wires:
  myu/1 -> Add/2
  Constant/1 -> Divide1/2
  Math Function1/1 -> Product1/1
  Divide1/1 -> Product2/1
  d2/1 -> Divide1/1, Product/3  "d2"
  Math Function2/1 -> Product3/2, Product1/2  "inv_cov"
  Product1/1 -> Product2/2
  d1/1 -> Product/2  "d1"
  x/1 -> Add/1
  Math Function/1 -> Product/4
  Product2/1 -> Math Function/1
  Add/1 -> Product1/3, Math Function1/1  "x-myu"
  sigma/1 -> Math Function2/1
  Product/1 -> jaco_add/3(num)
  index/1 -> jaco_add/2(index), gradient_col/1(index)
  jaco_add/1(jacobian) -> Out1/1
  set_jacobian/1 -> jaco_add/1("jacobian ")
  set_gradient/1 -> gradient_col/2(gradient)
  gradient_col/1(y) -> Product3/1
  data/1 -> Product4/1
  Product3/1 -> Product4/2
  Product4/1 -> Product/1

== system NDT_Localization/observation_callback/check_localizer/If Action Subsystem/register_measurement_impl/If Action Subsystem/If Action Subsystem/solve/If Action Subsystem1/For Iterator Subsystem/compute_next_step/If Action Subsystem1/For Iterator Subsystem/If Action Subsystem/If Action Subsystem3/If Action Subsystem/f_u/For Iterator Subsystem/make_c_param ==
  outlier_ratio : Inport
  voxel_size_x : Inport  Port=2
  voxel_size_y : Inport  Port=3
  voxel_size_z : Inport  Port=4
  Constant : Constant
  Divide : Product  Inputs=*/
  Gain : Gain  Gain=10
  Product : Product  Inputs=3
  Subtract : Sum  Inputs=+-
  c1 : Outport
  c2 : Outport  Port=2
  wires:
  Constant/1 -> Subtract/1
  outlier_ratio/1 -> Divide/1, Subtract/2
  Subtract/1 -> Gain/1
  Gain/1 -> c1/1
  Product/1 -> Divide/2
  Divide/1 -> c2/1
  voxel_size_y/1 -> Product/2
  voxel_size_z/1 -> Product/3
  voxel_size_x/1 -> Product/1

== system NDT_Localization/observation_callback/check_localizer/If Action Subsystem/register_measurement_impl/If Action Subsystem/If Action Subsystem/solve/If Action Subsystem1/For Iterator Subsystem/compute_next_step/If Action Subsystem1/For Iterator Subsystem/If Action Subsystem/If Action Subsystem3/If Action Subsystem/f_u/For Iterator Subsystem/make_d_param ==
  c1 : Inport
  c2 : Inport  Port=2
  Add1 : Sum
  Add2 : Sum  Inputs=-+
  Add3 : Sum
  Add4 : Sum  Inputs=+-
  Constant : Constant  Value=-2
  Constant1 : Constant  Value=-0.5
  Divide : Product  Inputs=*/
  Math Function{3..4,6..7} (4 alike) : Math  Operator=log
  Math Function5 : Math
  Product3 : Product
  Product4 : Product
  d1 : Outport
  d2 : Outport  Port=2
  wires:
  Add2/1 -> Divide/2, d1/1  "d1"
  Math Function4/1 -> Add4/1, Add2/2  "-d3"
  Product4/1 -> Add3/1
  Add3/1 -> Math Function6/1
  c1/1 -> Product4/1, Add1/1
  Constant/1 -> Product3/2
  Constant1/1 -> Math Function5/1
  Product3/1 -> d2/1  "d2"
  Math Function5/1 -> Product4/2
  Math Function7/1 -> Product3/1
  Divide/1 -> Math Function7/1
  Math Function6/1 -> Add4/2
  c2/1 -> Add3/2, Math Function4/1, Add1/2
  Add4/1 -> Divide/1
  Add1/1 -> Math Function3/1
  Math Function3/1 -> Add2/1
